simulink model "k1visprmp"  (Simulink 8.8)
settings: Solver=ode45  StartTime=0.0  StopTime=10.0  RelTol=1e-3  EnableMultiTasking=on
libraries: cdsIPCx x12, cdsCDI64 x3, cdsCDO64 x3, PAYLOAD_MASTER x3, dac x2, cdsAdcx0 x1, QPD x1, cdsParameters x1
settings Model: SuppressorTable=22 serialization::archive 11 0 3 0 0 0 11 0  Creator=keiko  LastModifiedBy=controls
settings DataIOCC: SignalLoggingSaveFormat=Dataset
settings DebuggingCC: UnderspecifiedInitializationDetection=Simplified  MergeDetectMultiDrivingBlocksExec=error  SolverPrmCheckMsg=warning  FcnCallInpInsideContextMsg=error  AllowSymbolicDim=off  StateNameClashWarn=none
settings GRTTargetCC: CombineOutputUpdateFcns=on  GRTInterface=off

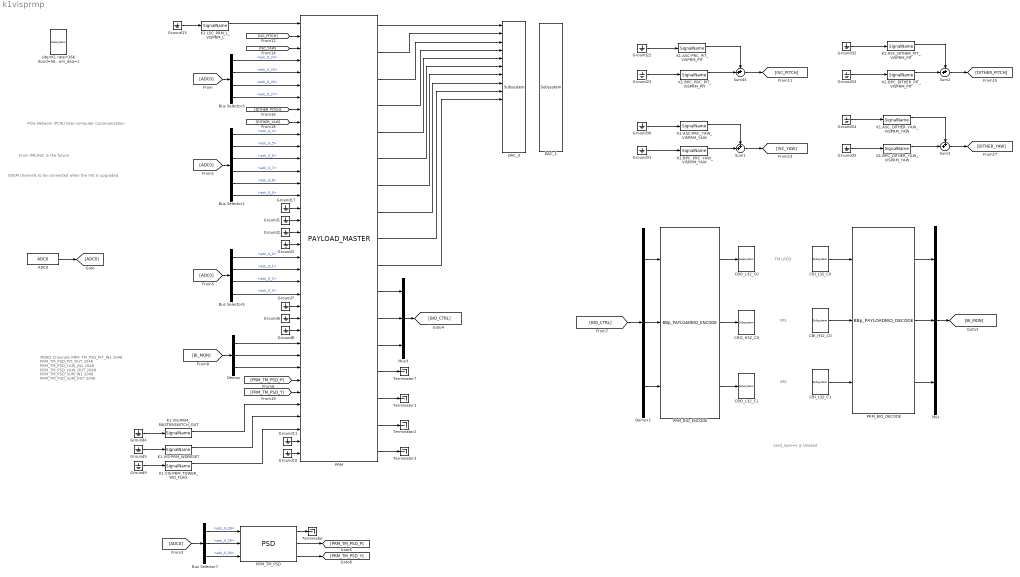
== system k1visprmp ==
  note: OSEM channels to be connected
      | when the VIS is upgraded.
  note: PCIe Network (PCIE)
      | Inter-computer Communication
  note: From IMCASC in the future.
  note: card_num=1 is Unused
  note: TM LPCD
  note: IM1
  note: IM2
  note: #DAQ Channels
      |
      | PRM_TM_PSD_PIT_IN1 2048
      | PRM_TM_PSD_PIT_OUT 2048
      | PRM_TM_PSD_YAW_IN1 2048
      | PRM_TM_PSD_YAW_OUT 2048
      | PRM_TM_PSD_SUM_IN1 2048
      | PRM_TM_PSD_SUM_OUT 2048
  ADC0 : cdsAdcx0/ADC0  Tag=cdsAdc  Description=|
      | type-GSC_16AI64SSA
      | card_num=0
      settings: AttributesFormatString=%<Description>\n%<Tag>
  Bus Selector1 : BusSelector  Description=ADC Selector  OutputSignals=adc_0_4,adc_0_5,adc_0_6,adc_0_7,adc_0_8,adc_0_9
      settings: AttributesFormatString=%<Description>
  Bus Selector3 : BusSelector  Description=ADC Selector  OutputSignals=adc_0_24,adc_0_25,adc_0_26,adc_0_27
      settings: AttributesFormatString=%<Description>
  Bus Selector5 : BusSelector  Description=ADC Selector  OutputSignals=adc_0_0,adc_0_1,adc_0_2,adc_0_3
      settings: AttributesFormatString=%<Description>
  Bus Selector7 : BusSelector  Description=ADC Selector  OutputSignals=adc_0_28,adc_0_29,adc_0_30
      settings: AttributesFormatString=%<Description>
  CBI_H32_C0 : cdsCDI64/Subsystem  Tag=cdsCDI64  Description=card_num=1
      settings: AttributesFormatString=%<Tag>\n%<Description>
  CBI_L32_C0 : cdsCDI64/Subsystem  Tag=cdsCDI64  Description=card_num=0
      settings: AttributesFormatString=%<Tag>\n%<Description>
  CBI_L32_C1 : cdsCDI64/Subsystem  Tag=cdsCDI64  Description=card_num=2
      settings: AttributesFormatString=%<Tag>\n%<Description>
  CBO_H32_C0 : cdsCDO64/Subsystem  Tag=cdsCDO64  Description=card_num=1
      settings: AttributesFormatString=%<Tag>\n%<Description>
  CBO_L32_C0 : cdsCDO64/Subsystem  Tag=cdsCDO64  Description=card_num=0
      settings: AttributesFormatString=%<Tag>\n%<Description>
  CBO_L32_C1 : cdsCDO64/Subsystem  Tag=cdsCDO64  Description=card_num=2
      settings: AttributesFormatString=%<Tag>\n%<Description>
  DAC_0 : dac/Subsystem  Description=|
      | type=GSC_16AO16,
      | card_num=0
      settings: AttributesFormatString=%<Description>
  DAC_1 : dac/Subsystem  Description=|
      | type=GSC_16AO16,
      | card_num=1
      settings: AttributesFormatString=%<Description>
  Demux : Demux  Outputs=3
  Demux1 : Demux  Outputs=3
  Ground{1..11,13,17,22..23,30..35} (21 alike) : Ground
  K1:ASC-PRC_PIT_VISPRM_PIT : cdsIPCx/SignalName  Tag=cdsIPCx_PCIE  Description=Inter-Process Communication via PCI Express network.
      settings: AttributesFormatString=%<Tag>
  K1:ASC-PRC_YAW_VISPRM_YAW : cdsIPCx/SignalName  Tag=cdsIPCx_PCIE  Description=Inter-Process Communication via PCI Express network.
      settings: AttributesFormatString=%<Tag>
  K1:ASC_DITHER_PIT_VISPRM_PIT : cdsIPCx/SignalName  Tag=cdsIPCx_PCIE  Description=Inter-Process Communication via PCI Express network.
      settings: AttributesFormatString=%<Tag>
  K1:ASC_DITHER_YAW_VISPRM_YAW : cdsIPCx/SignalName  Tag=cdsIPCx_PCIE  Description=Inter-Process Communication via PCI Express network.
      settings: AttributesFormatString=%<Tag>
  K1:BPC_DITHER_PIT_VISPRM_PIT : cdsIPCx/SignalName  Tag=cdsIPCx_PCIE  Description=Inter-Process Communication via PCI Express network.
      settings: AttributesFormatString=%<Tag>
  K1:BPC_DITHER_YAW_VISPRM_YAW : cdsIPCx/SignalName  Tag=cdsIPCx_PCIE  Description=Inter-Process Communication via PCI Express network.
      settings: AttributesFormatString=%<Tag>
  K1:BPC_PRC_PIT_VISPRM_PIT : cdsIPCx/SignalName  Tag=cdsIPCx_PCIE  Description=Inter-Process Communication via PCI Express network.
      settings: AttributesFormatString=%<Tag>
  K1:BPC_PRC_YAW_VISPRM_YAW : cdsIPCx/SignalName  Tag=cdsIPCx_PCIE  Description=Inter-Process Communication via PCI Express network.
      settings: AttributesFormatString=%<Tag>
  K1:LSC_PRM_L_VISPRM_L : cdsIPCx/SignalName  Tag=cdsIPCx_PCIE  Description=Inter-Process Communication via PCI Express network.
      settings: AttributesFormatString=%<Tag>
  K1:VIS-PRM_MASTERSWITCH_OUT : cdsIPCx/SignalName  Tag=cdsIPCx_SHMEM  Description=Inter-Process Communication via Shared memory.
      settings: AttributesFormatString=%<Tag>
  K1:VIS-PRM_TOWER_WD_FLAG : cdsIPCx/SignalName  Tag=cdsIPCx_SHMEM  Description=Inter-Process Communication via Shared memory.
      settings: AttributesFormatString=%<Tag>
  K1:VIS-PRM_WDRESET : cdsIPCx/SignalName  Tag=cdsIPCx_SHMEM  Description=Inter-Process Communication via Shared memory.
      settings: AttributesFormatString=%<Tag>
  Mux : Mux  Inputs=3
  Mux3 : Mux  Inputs=3
  PRM : PAYLOAD_MASTER/PAYLOAD_MASTER  Description=This is for Type-B and Bp payloads.
      settings: AttributesFormatString=%<Description>
  PRM_BIO_DECODE : PAYLOAD_MASTER/BBp_PAYLOADBIO_DECODE
  PRM_BIO_ENCODE : PAYLOAD_MASTER/BBp_PAYLOADBIO_ENCODE
  PRM_TM_PSD : QPD/PSD
  Sum{1..3,45} (4 alike) : Sum  Inputs=++|
  Terminator{,1..3,7} (5 alike) : Terminator
  site=K1 rate=16K dcuid=56 host=k1prm specific_cpu=3 adcSlave=1 shmem_daq=1 : cdsParameters/Subsystem  Tag=cdsParameters  Description=|
      | Purpose:                                                                                                                                                                                                                                
      | Provide system parameters to the FE code generator to properly configure the generated EPICS names, rep rate of the FE controller, and the Data Acquisition node ID for proper storage of data from this FE controller.                 
      |                                                                                                                                                                                                                                         
      | Useage:                                                                                                                                                                                                                                 
      | The part NAME field is used to identify the FE parameters. It must be of the form:                                                                                                                                                      
      | site=                                                                                                                                                                                                                                   
      | rate=                                                                                                                                                                                                                                   
      | dcuid=                                                                                                                                                                                                                                  
      |                                                                                                                                                                                                                                         
      | Where:                                                                                                                                                                                                                                  
      | site= argument may be H1, H2, L1, M1, G1, either as a single argument or multiple, for example site=H1,H2. These are the only names allowed. These will become the first two characters of all EPICS and signal names (for example G1:).
      |                                                                                                                                                                                                                                         
      | rate= may be 2K, 16K, 32K, or 64K                                                                                                                                                                                                       
      |                                                                                                                                                                                                                                         
      | dcuid= is site specific ie it must be unique at each site.
      settings: AttributesFormatString=%<Tag>
  wires:
  PRM/2 -> DAC_0/2
  PRM/3 -> DAC_0/3
  PRM/4 -> DAC_0/4
  PRM/1 -> DAC_0/1
  PRM/5 -> DAC_0/5
  PRM/6 -> DAC_0/6
  PRM/7 -> DAC_0/7
  PRM/8 -> DAC_0/8
  PRM/9 -> DAC_0/9
  PRM/10 -> DAC_0/10
  PRM/11 -> Mux3/1
  PRM/12 -> Mux3/2
  PRM/13 -> Mux3/3
  Mux3/1 -> [BIO_CTRL]
  PRM_BIO_DECODE/2 -> Mux/2
  PRM_BIO_DECODE/3 -> Mux/3
  PRM_BIO_DECODE/1 -> Mux/1
  Mux/1 -> [BI_MON]
  [BIO_CTRL] -> Demux1/1
  Demux1/1 -> PRM_BIO_ENCODE/1
  Demux1/2 -> PRM_BIO_ENCODE/2
  Demux1/3 -> PRM_BIO_ENCODE/3
  [ADC0] -> Bus Selector1/1
  K1:LSC_PRM_L_VISPRM_L/1 -> PRM/1
  Bus Selector1/1 -> PRM/10  "<adc_0_4>"
  [ADC0] -> Bus Selector7/1
  Bus Selector3/4 -> PRM/7  "<adc_0_27>"
  Bus Selector3/1 -> PRM/4  "<adc_0_24>"
  Bus Selector3/3 -> PRM/6  "<adc_0_26>"
  Bus Selector3/2 -> PRM/5  "<adc_0_25>"
  [ADC0] -> Bus Selector3/1
  Bus Selector1/2 -> PRM/11  "<adc_0_5>"
  Bus Selector1/3 -> PRM/12  "<adc_0_6>"
  Bus Selector1/4 -> PRM/13  "<adc_0_7>"
  Bus Selector1/5 -> PRM/14  "<adc_0_8>"
  Bus Selector1/6 -> PRM/15  "<adc_0_9>"
  Bus Selector5/2 -> PRM/21  "<adc_0_1>"
  Bus Selector5/3 -> PRM/22  "<adc_0_2>"
  Bus Selector5/4 -> PRM/23  "<adc_0_3>"
  [BI_MON] -> Demux/1
  Demux/1 -> PRM/27
  Demux/2 -> PRM/28
  Demux/3 -> PRM/29
  Ground8/1 -> PRM/26
  Ground6/1 -> PRM/25
  Ground7/1 -> PRM/24
  Bus Selector5/1 -> PRM/20  "<adc_0_0>"
  [ADC0] -> Bus Selector5/1
  ADC0/1 -> [ADC0]
  CBI_L32_C0/1 -> PRM_BIO_DECODE/1
  CBI_L32_C1/1 -> PRM_BIO_DECODE/3
  PRM_BIO_ENCODE/2 -> CBO_H32_C0/1
  PRM_BIO_ENCODE/3 -> CBO_L32_C1/1
  PRM_BIO_ENCODE/1 -> CBO_L32_C0/1
  CBI_H32_C0/1 -> PRM_BIO_DECODE/2
  Bus Selector7/1 -> PRM_TM_PSD/1  "<adc_0_28>"
  Bus Selector7/2 -> PRM_TM_PSD/2  "<adc_0_29>"
  Bus Selector7/3 -> PRM_TM_PSD/3  "<adc_0_30>"
  PRM_TM_PSD/1 -> Terminator/1
  PRM_TM_PSD/2 -> [PRM_TM_PSD_P]
  PRM_TM_PSD/3 -> [PRM_TM_PSD_Y]
  Ground13/1 -> K1:LSC_PRM_L_VISPRM_L/1
  Sum45/1 -> [ISC_PITCH]
  Ground22/1 -> K1:ASC-PRC_PIT_VISPRM_PIT/1
  Ground23/1 -> K1:BPC_PRC_PIT_VISPRM_PIT/1
  K1:ASC-PRC_PIT_VISPRM_PIT/1 -> Sum45/1
  K1:BPC_PRC_PIT_VISPRM_PIT/1 -> Sum45/2
  Sum1/1 -> [ISC_YAW]
  Sum2/1 -> [DITHER_PITCH]
  Sum3/1 -> [DITHER_YAW]
  Ground30/1 -> K1:ASC-PRC_YAW_VISPRM_YAW/1
  K1:ASC-PRC_YAW_VISPRM_YAW/1 -> Sum1/1
  K1:BPC_PRC_YAW_VISPRM_YAW/1 -> Sum1/2
  Ground31/1 -> K1:BPC_PRC_YAW_VISPRM_YAW/1
  Ground33/1 -> K1:BPC_DITHER_PIT_VISPRM_PIT/1
  K1:BPC_DITHER_PIT_VISPRM_PIT/1 -> Sum2/2
  Ground35/1 -> K1:BPC_DITHER_YAW_VISPRM_YAW/1
  K1:BPC_DITHER_YAW_VISPRM_YAW/1 -> Sum3/2
  K1:ASC_DITHER_PIT_VISPRM_PIT/1 -> Sum2/1
  Ground34/1 -> K1:ASC_DITHER_YAW_VISPRM_YAW/1
  Ground32/1 -> K1:ASC_DITHER_PIT_VISPRM_PIT/1
  K1:ASC_DITHER_YAW_VISPRM_YAW/1 -> Sum3/1
  [ISC_PITCH] -> PRM/2
  [ISC_YAW] -> PRM/3
  [DITHER_PITCH] -> PRM/8
  [DITHER_YAW] -> PRM/9
  [PRM_TM_PSD_Y] -> PRM/31
  [PRM_TM_PSD_P] -> PRM/30
  Ground17/1 -> PRM/16
  Ground1/1 -> PRM/17
  Ground2/1 -> PRM/18
  Ground3/1 -> PRM/19
  Ground4/1 -> K1:VIS-PRM_MASTERSWITCH_OUT/1
  K1:VIS-PRM_MASTERSWITCH_OUT/1 -> PRM/32
  K1:VIS-PRM_WDRESET/1 -> PRM/33
  Ground5/1 -> K1:VIS-PRM_WDRESET/1
  K1:VIS-PRM_TOWER_WD_FLAG/1 -> PRM/34
  Ground9/1 -> K1:VIS-PRM_TOWER_WD_FLAG/1
  PRM/14 -> Terminator7/1
  PRM/15 -> Terminator1/1
  PRM/16 -> Terminator2/1
  Ground11/1 -> PRM/35
  Ground10/1 -> PRM/36
  PRM/17 -> Terminator3/1
